simulink model "teste_solenoide_PWM_Final"  (R2023a)
settings: Solver=VariableStepAuto  StartTime=0.0  StopTime=11  RelTol=1e-3
libraries: fl_lib x15, nesl_utility x7, spsMeanLib x6, SimscapeFluids_lib x6, simulink x1
settings Model: Creator=Nautec  LastModifiedBy=nautec-01
settings HardwareCC: ProdBitPerLong=64  ProdHWDeviceType=Apple->ARM64

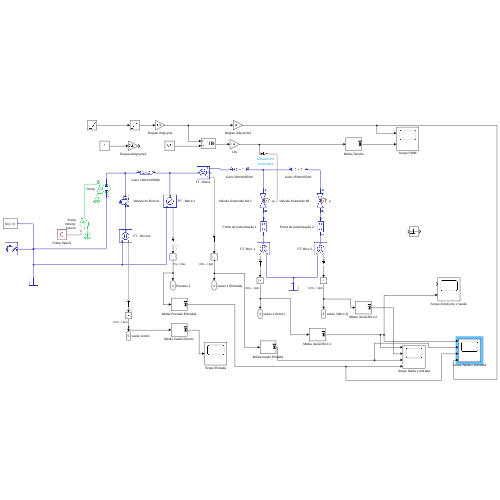
[thumbnail: Simulink's stored preview of the top-level diagram]
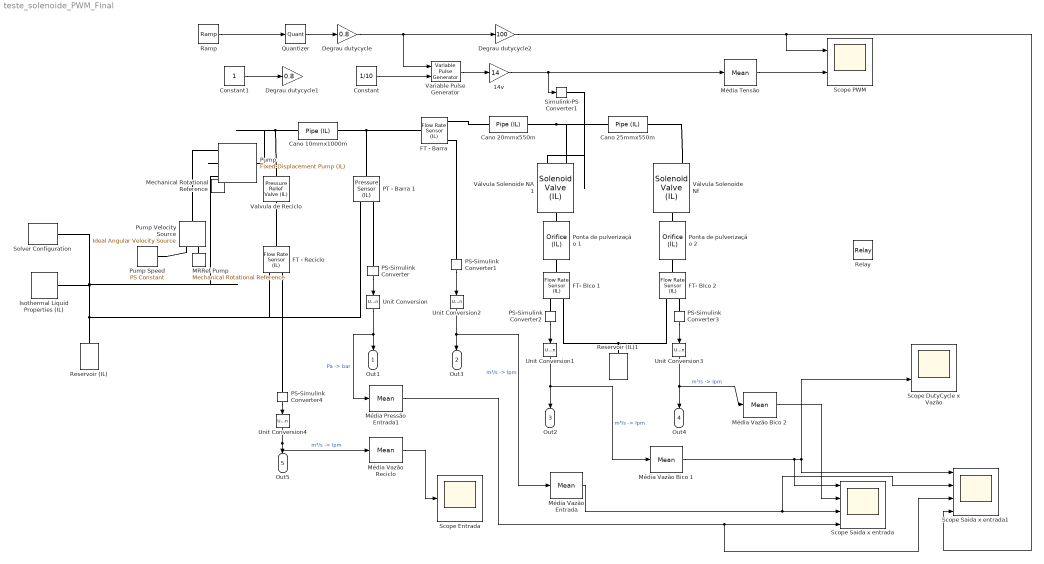
== system teste_solenoide_PWM_Final ==
  14v : Gain  Gain=14
  Cano 10mmx1000m : fl_lib/Isothermal Liquid/Elements/Pipe (IL)  length=1 m  area=78.53 mm^2  Dh=10 mm  length_add=1 m  roughness=15e-6 m  Re_lam=2000  Re_tur=4000  shape_factor=64  dynamic_compressibility=simscape.enum.onoff.on  inertia=simscape.enum.onoff.off  p0=0.101325 MPa  mdot0=0 kg/s
      settings: InternalSimscapePortConfiguration="{\"Bottom\":[],\"Left\":[{\"id\":\"A\",\"label\":\"A\",\"type\":\"foundation.isothermal_liquid.isothermal_liquid\"}],\"Right\":[{\"id\":\"B\",\"label\":\"B\",\"type\":\"foundation.isothermal_liquid.isothermal_liquid\"}],\"Top\":[]}"
  Cano 20mmx550m : fl_lib/Isothermal Liquid/Elements/Pipe (IL)  length=55 mm  area=31415 mm^2  Dh=20 mm  length_add=1 m  roughness=15e-6 m  Re_lam=2000  Re_tur=4000  shape_factor=64  dynamic_compressibility=simscape.enum.onoff.on  inertia=simscape.enum.onoff.off  p0=0.101325 MPa  mdot0=0 kg/s
      settings: InternalSimscapePortConfiguration="{\"Bottom\":[],\"Left\":[{\"id\":\"A\",\"label\":\"A\",\"type\":\"foundation.isothermal_liquid.isothermal_liquid\"}],\"Right\":[{\"id\":\"B\",\"label\":\"B\",\"type\":\"foundation.isothermal_liquid.isothermal_liquid\"}],\"Top\":[]}"
  Cano 25mmx550m : fl_lib/Isothermal Liquid/Elements/Pipe (IL)  length=55 mm  area=49087 mm^2  Dh=25 mm  length_add=1 m  roughness=15e-6 m  Re_lam=2000  Re_tur=4000  shape_factor=64  dynamic_compressibility=simscape.enum.onoff.on  inertia=simscape.enum.onoff.off  p0=0.101325 MPa  mdot0=0 kg/s
      settings: InternalSimscapePortConfiguration="{\"Bottom\":[],\"Left\":[{\"id\":\"A\",\"label\":\"A\",\"type\":\"foundation.isothermal_liquid.isothermal_liquid\"}],\"Right\":[{\"id\":\"B\",\"label\":\"B\",\"type\":\"foundation.isothermal_liquid.isothermal_liquid\"}],\"Top\":[]}"
  Constant : Constant  Value=1/10
  Constant1 : Constant
  Degrau dutycycle : Gain  Gain=0.8
  Degrau dutycycle1 : Gain  Gain=0.8
  Degrau dutycycle2 : Gain  Gain=100
  FT - Barra : fl_lib/Isothermal Liquid/Sensors/Flow Rate Sensor (IL)  sensor_type=foundation.enum.mass_volumetric_sensor.mass_volumetric
      settings: InternalSimscapePortConfiguration="{\"Bottom\":[],\"Left\":[{\"id\":\"A\",\"label\":\"A\",\"type\":\"foundation.isothermal_liquid.isothermal_liquid\"}],\"Right\":[{\"id\":\"B\",\"label\":\"B\",\"type\":\"foundation.isothermal_liquid.isothermal_liquid\"},{\"id\":\"M\",\"label\":\"M\",\"type\":\"output\"},{\"id\":\"V\",\"label\":\"V\",\"type\":\"output\"}],\"Top\":[]}"
  FT - Reciclo : fl_lib/Isothermal Liquid/Sensors/Flow Rate Sensor (IL)  sensor_type=foundation.enum.mass_volumetric_sensor.volumetric
      settings: InternalSimscapePortConfiguration="{\"Bottom\":[],\"Left\":[{\"id\":\"A\",\"label\":\"A\",\"type\":\"foundation.isothermal_liquid.isothermal_liquid\"}],\"Right\":[{\"id\":\"B\",\"label\":\"B\",\"type\":\"foundation.isothermal_liquid.isothermal_liquid\"},{\"id\":\"V\",\"label\":\"V\",\"type\":\"output\"}],\"Top\":[]}"
  FT- BIco 1 : fl_lib/Isothermal Liquid/Sensors/Flow Rate Sensor (IL)  sensor_type=foundation.enum.mass_volumetric_sensor.volumetric
      settings: InternalSimscapePortConfiguration="{\"Bottom\":[],\"Left\":[{\"id\":\"A\",\"label\":\"A\",\"type\":\"foundation.isothermal_liquid.isothermal_liquid\"}],\"Right\":[{\"id\":\"B\",\"label\":\"B\",\"type\":\"foundation.isothermal_liquid.isothermal_liquid\"},{\"id\":\"V\",\"label\":\"V\",\"type\":\"output\"}],\"Top\":[]}"
  FT- BIco 2 : fl_lib/Isothermal Liquid/Sensors/Flow Rate Sensor (IL)  sensor_type=foundation.enum.mass_volumetric_sensor.volumetric
      settings: InternalSimscapePortConfiguration="{\"Bottom\":[],\"Left\":[{\"id\":\"A\",\"label\":\"A\",\"type\":\"foundation.isothermal_liquid.isothermal_liquid\"}],\"Right\":[{\"id\":\"B\",\"label\":\"B\",\"type\":\"foundation.isothermal_liquid.isothermal_liquid\"},{\"id\":\"V\",\"label\":\"V\",\"type\":\"output\"}],\"Top\":[]}"
  Isothermal Liquid Properties (IL) : fl_lib/Isothermal Liquid/Utilities/Isothermal Liquid Properties (IL)  rho_L_atm=998.21 kg/m^3  bulk_modulus_model=foundation.enum.bulk_modulus_model.const  beta_gain=6  beta_L_atm=2.1791e9 Pa  nu_atm=1.0034e-6 m^2/s  p_atm=0.101325 MPa  p_min=1 Pa  properties_range_check=simscape.enum.assert.action.error  air_fraction=0.005  polytropic_index=1.0  rho_g_atm=1.225 kg/m^3  air_dissolution_model=simscape.enum.onoff.off  p_crit=3 MPa
  MRRef Pump : fl_lib/Mechanical/Rotational Elements/Mechanical Rotational Reference  Tag=Factory Generic
  Mechanical Rotational Reference : fl_lib/Mechanical/Rotational Elements/Mechanical Rotational Reference
  Média Pressão Entrada1 : spsMeanLib/Mean  Freq=5  Vinit=0  Ts=0
  Média Tensão : spsMeanLib/Mean  Freq=10  Vinit=0  Ts=0
  Média Vazão Bico 1 : spsMeanLib/Mean  Freq=5  Vinit=0  Ts=0
  Média Vazão Bico 2 : spsMeanLib/Mean  Freq=5  Vinit=0  Ts=0
  Média Vazão Entrada : spsMeanLib/Mean  Freq=5  Vinit=0  Ts=0
  Média Vazão Reciclo : spsMeanLib/Mean  Freq=5  Vinit=0  Ts=0
  PS-Simulink Converter{,1..4} (5 alike) : nesl_utility/PS-Simulink Converter  PhysicalDomain=network_engine_domain  SubClassName=ps_output  LeftPortType=input  RightPortType=output  PseudoPeriodic=off  Frequencies=[]  VectorFormat=inherit  Unit=inherit  AffineConversion=off
  PT - Barra 1 : fl_lib/Isothermal Liquid/Sensors/Pressure Sensor (IL)  pressure_measure=foundation.enum.pressure_measure.difference
      settings: InternalSimscapePortConfiguration="{\"Bottom\":[],\"Left\":[{\"id\":\"A\",\"label\":\"A\",\"type\":\"foundation.isothermal_liquid.isothermal_liquid\"}],\"Right\":[{\"id\":\"B\",\"label\":\"B\",\"type\":\"foundation.isothermal_liquid.isothermal_liquid\"},{\"id\":\"P\",\"label\":\"P\",\"type\":\"output\"}],\"Top\":[]}"
  Ponta de pulverização 1 : SimscapeFluids_lib/Isothermal Liquid/Valves & Orifices/Orifices/Orifice (IL)  orifice_type=foundation.enum.constant_variable.constant  constant_orifice_spec=fluids.isothermal_liquid.valves_orifices.orifices.enum.constant_orifice_spec.area  variable_orifice_spec=fluids.isothermal_liquid.valves_orifices.orifices.enum.orifice_spec.linear  orifice_area_constant=0.5794 mm^2  p_diff_TLU_constant=[-4, -3, -2, -1, -.5, 0, .5, 1, 2, 3, 4] MPa  vol_flow_TLU_constant=[-2.44, -2.12, -1.68, -1.22, -.84, 0, .85, 1.21, 1.7, 2.09, 2.41] .* 1e-3 m^3/s  S_min=0 m  del_S=5e-3 m  open_orientation=fluids.isothermal_liquid.valves_orifices.orifices.enum.orifice_orientation.positive  area_max=1e-4 m^2  area_leak=1e-10 m^2  S_TLU=[0, .002, .004, .007, .017] m  orifice_area_TLU=[1e-09, 2.0352e-07, 4.0736e-05, .00011438, .00034356] m^2  area=inf m^2  Cd=0.7  Re_c=12  smoothing_factor=0.01  pressure_recovery=false  S_vol_flow_TLU=[0, .002, .004, .007, .017] m  p_diff_TLU=[.3, .5, .7] MPa  vol_flow_TLU=1e-3 * [1.7e-05, 2e-05, 2.6e-05; .0035, .0045, .0053; .7, .9, 1.06; 1.96, 2.5, 3; 6, 7.7, 9.13] m^3/s  enable_faults=simscape.enum.onoff.off  fault_action=fluids.enum.FaultOpening.Closed  external_fault=fluids.enum.FaultExternalTrigger.Off  temporal_fault=simscape.enum.onoff.off  fault_time=5 s  report_fault=simscape.enum.assert.action.none
      settings: InternalSimscapePortConfiguration="{\"Bottom\":[],\"Left\":[{\"id\":\"A\",\"label\":\"A\",\"type\":\"foundation.isothermal_liquid.isothermal_liquid\"}],\"Right\":[{\"id\":\"B\",\"label\":\"B\",\"type\":\"foundation.isothermal_liquid.isothermal_liquid\"}],\"Top\":[]}"
  Ponta de pulverização 2 : SimscapeFluids_lib/Isothermal Liquid/Valves & Orifices/Orifices/Orifice (IL)  orifice_type=foundation.enum.constant_variable.constant  constant_orifice_spec=fluids.isothermal_liquid.valves_orifices.orifices.enum.constant_orifice_spec.area  variable_orifice_spec=fluids.isothermal_liquid.valves_orifices.orifices.enum.orifice_spec.linear  orifice_area_constant=0.583 mm^2  p_diff_TLU_constant=[-4, -3, -2, -1, -.5, 0, .5, 1, 2, 3, 4] MPa  vol_flow_TLU_constant=[-2.44, -2.12, -1.68, -1.22, -.84, 0, .85, 1.21, 1.7, 2.09, 2.41] .* 1e-3 m^3/s  S_min=0 m  del_S=5e-3 m  open_orientation=fluids.isothermal_liquid.valves_orifices.orifices.enum.orifice_orientation.positive  area_max=1e-4 m^2  area_leak=1e-10 m^2  S_TLU=[0, .002, .004, .007, .017] m  orifice_area_TLU=[1e-09, 2.0352e-07, 4.0736e-05, .00011438, .00034356] m^2  area=inf m^2  Cd=0.7  Re_c=12  smoothing_factor=0.01  pressure_recovery=false  S_vol_flow_TLU=[0, .002, .004, .007, .017] m  p_diff_TLU=[.3, .5, .7] MPa  vol_flow_TLU=1e-3 * [1.7e-05, 2e-05, 2.6e-05; .0035, .0045, .0053; .7, .9, 1.06; 1.96, 2.5, 3; 6, 7.7, 9.13] m^3/s  enable_faults=simscape.enum.onoff.off  fault_action=fluids.enum.FaultOpening.Closed  external_fault=fluids.enum.FaultExternalTrigger.Off  temporal_fault=simscape.enum.onoff.off  fault_time=5 s  report_fault=simscape.enum.assert.action.none
      settings: InternalSimscapePortConfiguration="{\"Bottom\":[],\"Left\":[{\"id\":\"A\",\"label\":\"A\",\"type\":\"foundation.isothermal_liquid.isothermal_liquid\"}],\"Right\":[{\"id\":\"B\",\"label\":\"B\",\"type\":\"foundation.isothermal_liquid.isothermal_liquid\"}],\"Top\":[]}"
  Pump : SimscapeFluids_lib/Isothermal Liquid/Pumps & Motors/Fixed-Displacement Pump (IL)  Tag=Factory Generic  leakage_friction_spec=fluids.isothermal_liquid.pumps_motors.enum.pump_motor_loss_spec.analytical  displacement=5.5/1200 l/rev  omega_nominal=550 rpm  p_nominal=9 bar  vol_eff_nominal=0.92  mech_eff_nominal=0.8695652173913044  no_load_torque=0 N*m  p_diff_eff_TLU=[100000.0, 1000000.0, 2000000.0] Pa  omega_eff_TLU=[25.0, 50.0, 100.0, 200.0, 300.0, 400.0] rad/s  vol_eff_TLU=[0.816, 0.908, 0.954, 0.977, 0.981, 0.984; 0.325, 0.663, 0.831, 0.916, 0.925, 0.946; 0.137, 0.568, 0.78, 0.892, 0.893, 0.91]  mech_eff_TLU=[0.996, 0.996, 0.996, 0.996, 0.996, 0.996; 0.988, 0.989, 0.989, 0.989, 0.989, 0.99; 0.981, 0.981, 0.982, 0.982, 0.983, 0.984]  p_diff_loss_TLU=[100000.0, 1000000.0, 2000000.0] Pa  omega_loss_TLU=[25.0, 50.0, 100.0, 200.0, 300.0, 400.0] rad/s  vol_loss_TLU=[0.023, 0.023, 0.023, 0.023, 0.0285, 0.032; 0.0844, 0.0842, 0.0845, 0.084, 0.1125, 0.108; 0.1079, 0.108, 0.11, 0.108, 0.1605, 0.18] * 1e-3 m^3/s  mech_loss_TLU=[0.002, 0.002, 0.002, 0.002, 0.002, 0.002; 0.0607, 0.0556, 0.0556, 0.0556, 0.0556, 0.0505; 0.1937, 0.1937, 0.1833, 0.1833, 0.1729, 0.1626] N*m  vol_eff_min=1e-3  vol_eff_max=1  mech_eff_min=1e-3  mech_eff_max=1  pressure_threshold=1e5 Pa  omega_threshold=10 rad/s  quadrant_check=simscape.enum.assert.action.none  pump_mode_check=simscape.enum.assert.action.none  pressure_check=simscape.enum.assert.action.none  p_min_valid=0 + 101325 Pa
      settings: InternalSimscapePortConfiguration="{\"Bottom\":[{\"id\":\"A\",\"label\":\"A\",\"type\":\"foundation.isothermal_liquid.isothermal_liquid\"}],\"Left\":[],\"Right\":[{\"id\":\"R\",\"label\":\"R\",\"type\":\"foundation.mechanical.rotational.rotational\"},{\"id\":\"C\",\"label\":\"C\",\"type\":\"foundation.mechanical.rotational.rotational\"}],\"Top\":[{\"id\":\"B\",\"label\":\"B\",\"type\":\"foundation.isothermal_liquid.isothermal_liquid\"}]}"
  Pump Velocity Source : fl_lib/Mechanical/Mechanical Sources/Ideal Angular Velocity Source  Tag=Factory Generic
  Pump Speed : fl_lib/Physical Signals/Sources/PS Constant  constant=780/60*2*pi
  Quantizer : Quantizer  QuantizationInterval=0.1
  Ramp : simulink/Sources/Ramp  slope=0.1  start=0  InitialOutput=0
  Relay : Relay
  Reservoir (IL) : fl_lib/Isothermal Liquid/Elements/Reservoir (IL)  reservoir_type=foundation.enum.constant_controlled.constant  pressure_spec=foundation.enum.pressure_spec.atmospheric  reservoir_pressure=0.101325 MPa
  Reservoir (IL)1 : fl_lib/Isothermal Liquid/Elements/Reservoir (IL)  reservoir_type=foundation.enum.constant_controlled.constant  pressure_spec=foundation.enum.pressure_spec.atmospheric  reservoir_pressure=0.101325 MPa
  Scope DutyCycle x Vazão : Scope  NumInputPorts=2
  Scope Entrada : Scope
  Scope PWM : Scope  NumInputPorts=2
  Scope Saida x entrada : Scope  NumInputPorts=4
  Scope Saida x entrada1 : Scope  NumInputPorts=4
  Simulink-PS Converter1 : nesl_utility/Simulink-PS Converter  PhysicalDomain=network_engine_domain  SubClassName=ps_input  LeftPortType=input  RightPortType=output  PseudoPeriodic=off  Frequencies=[]  NoiseDistribution=none  NoiseParameters=[]  Unit=1  AffineConversion=off  FilteringAndDerivatives=provide  SimscapeFilterOrder=1  InputFilterTimeConstant=0.001  UdotUserProvided=0
  Solver Configuration : nesl_utility/Solver Configuration  PhysicalDomain=network_engine_domain  SubClassName=solver  LeftPortType=input  RightPortType=generic  Tones=[]  Harmonics=[]  SimulateNoise=off  Profile=off  UseLocalSampling=off  EnableSwitchedLinearOptims=on  FrequencyDomain=off  UseCCode=off  RelTol=0.001  AbsTol=0.001  MinStep=1e-09  ToWorkspace=off  RevertToSquareIcSolve=off  NumHomotopyIterations=100  PhasorMode=off  PhasorModeNumHarmonics=1  ConsistencySolver=NEWTON_XTOL_AFTER_FTOL  IndexReductionMethod=DerivativeReplacement  DoDC=off  ResidualTolerance=1e-09  ConsistencyTolSource=GLOBAL  ConsistencyAbsTol=0.001  ConsistencyRelTol=0.001  ConsistencyTolFactor=0.001  UseLocalSolver=off  LocalSolverChoice=NE_BACKWARD_EULER_ADVANCER  ResolveIndetEquations=on  FunctionEvalNumThread=1  LocalSolverSampleTime=0.001  DoFixedCost=off  MaxNonlinIter=3  MaxModeIter=2  ComputeImpulses=off  ImpulseIterations=2  LinearAlgebra=auto  LinearAlgebraNumThread=0  EquationFormulation=NE_TIME_EF  DelaysMemoryBudget=1024  AutomaticFiltering=on  FilteringTimeConstant=0.001  PartitionStorageMethod=AS_NEEDED  PartitionMemoryBudget=1024  PartitionMethod=ROBUST
  Unit Conversion{,1..4} (5 alike) : UnitConversion
  Valvula de Reciclo : SimscapeFluids_lib/Isothermal Liquid/Valves & Orifices/Pressure Control Valves/Pressure Relief Valve (IL)  set_pressure_spec=foundation.enum.constant_controlled.constant  opening_spec=fluids.isothermal_liquid.valves_orifices.enum.PressureOpeningSpec.Linear  pressure_spec=fluids.isothermal_liquid.valves_orifices.enum.pressure_control_spec.dp  p_set_gauge=0.1 MPa  p_set_differential=2 bar  p_range=0.1 bar  area_max=1e-4 m^2  area_leak=1e-10 m^2  p_diff_TLU=[0.2 : 0.2 : 1.2] MPa  p_gauge_TLU=[0.2 : 0.2 : 1.2] MPa  valve_area_TLU=[1e-10, 2e-06, 4e-06, 6e-06, 8e-06, 1e-05] m^2  vol_flow_TLU=[1e-09, 3.6e-05, 8.9e-05, .00015, .00023, .00031] m^3/s  area=inf m^2  Cd=0.64  Re_c=150  smoothing_factor=0.01  pressure_recovery=false  opening_dynamics=false  tau=0.1 s  enable_faults=simscape.enum.onoff.off  fault_type=fluids.enum.FaultOpening.Closed  fault_trigger=foundation.enum.faultSpec.Temporal  fault_time=5 s
      settings: InternalSimscapePortConfiguration="{\"Bottom\":[],\"Left\":[{\"id\":\"A\",\"label\":\"A\",\"type\":\"foundation.isothermal_liquid.isothermal_liquid\"}],\"Right\":[{\"id\":\"B\",\"label\":\"B\",\"type\":\"foundation.isothermal_liquid.isothermal_liquid\"}],\"Top\":[]}"
  Variable Pulse Generator : VariablePulseGenerator  AllowZeroPulseWidth=on  SampleTime=0.1
  Válvula Solenoide NA 1 : SimscapeFluids_lib/Isothermal Liquid/Valves & Orifices/Directional Control Valves/Solenoid Valve (IL)  init_position=fluids.isothermal_liquid.valves_orifices.enum.InitOpenClosedSpec.Open  open_switch_time=12.29 ms  close_switch_time=18.66 ms  area_max=72 mm^2  area_leak=1e-9 m^2  area=506 mm^2  Cd=0.64  Re_c=12  pressure_recovery=false
      settings: InternalSimscapePortConfiguration="{\"Bottom\":[],\"Left\":[{\"id\":\"A\",\"label\":\"A\",\"type\":\"foundation.isothermal_liquid.isothermal_liquid\"}],\"Right\":[{\"id\":\"B\",\"label\":\"B\",\"type\":\"foundation.isothermal_liquid.isothermal_liquid\"}],\"Top\":[{\"id\":\"S\",\"label\":\"S\",\"type\":\"input\"}]}"
  Válvula Solenoide Nf : SimscapeFluids_lib/Isothermal Liquid/Valves & Orifices/Directional Control Valves/Solenoid Valve (IL)  init_position=fluids.isothermal_liquid.valves_orifices.enum.InitOpenClosedSpec.Closed  open_switch_time=47.5 ms  close_switch_time=15.5 ms  area_max=72 mm^2  area_leak=1e-9 m^2  area=506 mm^2  Cd=0.64  Re_c=12  pressure_recovery=false
      settings: InternalSimscapePortConfiguration="{\"Bottom\":[],\"Left\":[{\"id\":\"A\",\"label\":\"A\",\"type\":\"foundation.isothermal_liquid.isothermal_liquid\"}],\"Right\":[{\"id\":\"B\",\"label\":\"B\",\"type\":\"foundation.isothermal_liquid.isothermal_liquid\"}],\"Top\":[{\"id\":\"S\",\"label\":\"S\",\"type\":\"input\"}]}"
  Out1 : Outport  SignalName=Pressao 1  Unit=bar
  Out3 : Outport  Port=2  SignalName=vazao 1 (Entrada)  Unit=l/min
  Out2 : Outport  Port=3  SignalName=vazao 2 (bico1)  Unit=l/min
  Out4 : Outport  Port=4  SignalName=vazao 3(bico 2)  Unit=l/min
  Out5 : Outport  Port=5  SignalName=vazao reciclo  Unit=lpm
  wires:
  Unit Conversion/1 -> Média Pressão Entrada1/1, Out1/1  "Pa -> bar"
  PS-Simulink Converter/1 -> Unit Conversion/1
  Unit Conversion2/1 -> Média Vazão Entrada/1, Out3/1  "m³/s -> lpm"
  PS-Simulink Converter1/1 -> Unit Conversion2/1
  PS-Simulink Converter2/1 -> Unit Conversion1/1
  Unit Conversion1/1 -> Média Vazão Bico 1/1, Out2/1  "m³/s -> lpm"
  PS-Simulink Converter3/1 -> Unit Conversion3/1
  Unit Conversion3/1 -> Out4/1, Média Vazão Bico 2/1  "m³/s -> lpm"
  PS-Simulink Converter4/1 -> Unit Conversion4/1
  Unit Conversion4/1 -> Média Vazão Reciclo/1, Out5/1  "m³/s -> lpm"
  Média Vazão Reciclo/1 -> Scope Entrada/1
  Constant/1 -> Variable Pulse Generator/2
  Variable Pulse Generator/1 -> 14v/1
  Quantizer/1 -> Degrau dutycycle/1
  Média Tensão/1 -> Scope PWM/2
  Média Vazão Bico 1/1 -> Scope Saida x entrada/1, Scope DutyCycle x Vazão/2, Scope Saida x entrada1/1
  Média Vazão Entrada/1 -> Scope Saida x entrada1/2, Scope Saida x entrada/3
  Média Pressão Entrada1/1 -> Scope Saida x entrada1/3, Scope Saida x entrada/4
  Constant1/1 -> Degrau dutycycle1/1
  Média Vazão Bico 2/1 -> Scope Saida x entrada/2
  Degrau dutycycle2/1 -> Scope PWM/1, Scope Saida x entrada1/4
  Degrau dutycycle/1 -> Degrau dutycycle2/1, Variable Pulse Generator/1
  Ramp/1 -> Quantizer/1
  14v/1 -> Simulink-PS Converter1/1, Média Tensão/1
  connections:
  Pump Speed/RConn1 -- Pump Velocity Source/RConn1
  Pump/RConn2 -- Mechanical Rotational Reference/LConn1
  Pump Velocity Source/LConn1 -- Pump/RConn1
  Pump Velocity Source/RConn2 -- MRRef Pump/LConn1
  Reservoir (IL)/LConn1 -- PT - Barra 1/RConn1 -- FT - Reciclo/RConn1 -- Isothermal Liquid Properties (IL)/RConn1 -- Solver Configuration/RConn1 -- Pump/RConn3
  PT - Barra 1/LConn1 -- FT - Barra/LConn1 -- Cano 10mmx1000m/RConn1
  PS-Simulink Converter2/LConn1 -- FT- BIco 1/RConn2
  PS-Simulink Converter3/LConn1 -- FT- BIco 2/RConn2
  FT - Reciclo/LConn1 -- Valvula de Reciclo/RConn1
  PT - Barra 1/RConn2 -- PS-Simulink Converter/LConn1
  Reservoir (IL)1/LConn1 -- FT- BIco 2/RConn1 -- FT- BIco 1/RConn1
  Ponta de pulverização 1/LConn1 -- Válvula Solenoide NA 1/RConn1
  Ponta de pulverização 1/RConn1 -- FT- BIco 1/LConn1
  Válvula Solenoide Nf/RConn1 -- Ponta de pulverização 2/LConn1
  Ponta de pulverização 2/RConn1 -- FT- BIco 2/LConn1
  PS-Simulink Converter4/LConn1 -- FT - Reciclo/RConn2
  Cano 10mmx1000m/LConn1 -- Valvula de Reciclo/LConn1 -- Pump/LConn1
  FT - Barra/RConn1 -- Cano 20mmx550m/LConn1
  Cano 25mmx550m/LConn1 -- Cano 20mmx550m/RConn1 -- Válvula Solenoide NA 1/LConn1
  Válvula Solenoide Nf/LConn1 -- Cano 25mmx550m/RConn1
  FT - Barra/RConn3 -- PS-Simulink Converter1/LConn1
  Simulink-PS Converter1/RConn1 -- Válvula Solenoide NA 1/LConn2
